simulink model "FuzzyControl"  (Simulink 8.9)
settings: Solver=FixedStepDiscrete  StartTime=0.0  StopTime=inf  FixedStep=0.002  RelTol=1e-3  EnableMultiTasking=on
undefined symbols (not defined in the file or in its folder): DiscIntNeverNeededParam, HIL
libraries: quarc_library x8, fuzblock x1
Description:
  | This example is a simple analog loopback test. It sends a signal to analog output
  | channel #0 and then reads analog input channel #0. Wire analog output #0 to analog
  | input #0 to see the signal on the Scope. Change the amplitude of the signal and see
  | the change occur on the Scope.
settings Model: Creator=drmadill  LastModifiedBy=yettbh  SimulationMode=external  ExtModeTrigDuration=10000
settings SolverCC: PositivePriorityOrder=on
settings OptimizationCC: ExpressionDepthLimit=2147483647  InitFltsAndDblsToZero=on  LifeSpan=auto
settings DebuggingCC: SaveWithParameterizedLinksMsg=none  SolverPrmCheckMsg=warning
settings RTWCC: SystemTargetFile=quarc_win64.tlc  TemplateMakefile=quarc_default_tmf  Description=QUARC Win64 Target
settings STFCustomTargetCC: TargetPreCompLibLocation=C:\PROGRA~3\QUARC\lib\2017a\win64\release  ConcurrentExecutionCompliant=on  SystemTargetFile=quarc_win64.tlc
settings GRTTargetCC: TargetPreCompLibLocation=C:\PROGRA~3\QUARC\lib\2017a\win64\release  ParMdlRefBuildCompliant=off  CompOptLevelCompliant=off  GeneratePreprocessorConditionals=Use local settings  MatFileLogging=off  CPPClassGenCompliant=off  UseToolchainInfoCompliant=off  ExtMode=on  ExtModeMexFile=quarc_comm

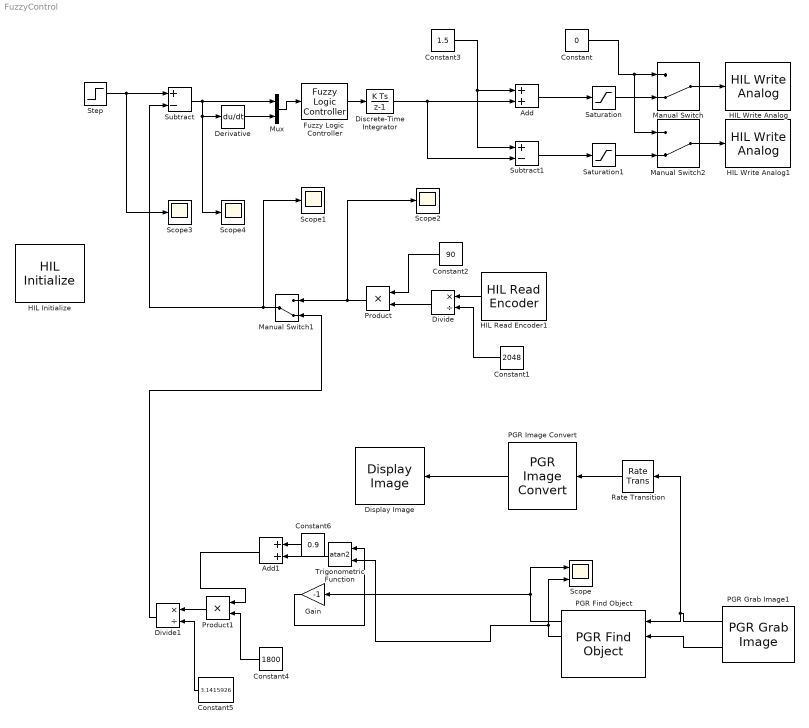
== system FuzzyControl ==
  Add : Sum
  Add1 : Sum
  Constant : Constant  Value=0
  Constant1 : Constant  Value=2048
  Constant2 : Constant  Value=90
  Constant3 : Constant  Value=1.5
  Constant4 : Constant  Value=1800
  Constant5 : Constant  Value=3.1415926
  Constant6 : Constant  Value=0.9
  Derivative : Derivative
  Discrete-Time Integrator : DiscreteIntegrator  SampleTime=0.002  ICPrevOutput=DiscIntNeverNeededParam  ICPrevScaledInput=DiscIntNeverNeededParam
  Display Image : quarc_library/Sinks/Figures/Display Image  figure_mode=Use figure window  figure_tag=figure1  axes_tag=axes1  update_rate=1  initial_position="48  432  563  457"  initial_visibility=off  sample_time=0.1  axes_only=off  orig_size=off
      settings: SourceProductName=QUARC Targets
  Divide : Product  Inputs=*/
  Divide1 : Product  Inputs=*/
  Fuzzy Logic  Controller : fuzblock/Fuzzy Logic  Controller  fis='vision.fis'
  Gain : Gain  Gain=-1
  HIL Initialize : quarc_library/Data Acquisition/Generic/Configuration/HIL Initialize  object_name=HIL-1  board_type=q8  board_number=0  board_options=""  exclusive=off  active=on  hardware_clocks=[0:1]  clock_modes=[0 0]  initial_clock_frequencies=[]  set_clock_params_at_start=on  set_clock_params_at_switch_in=off  set_clock_frequencies_at_start=off  set_clock_frequencies_at_switch_in=off  analog_input_channels=[0:7]  analog_input_configurations=[]  analog_input_maximums=10  analog_input_minimums=-10  set_analog_input_params_at_start=off  set_analog_input_params_at_switch_in=off  analog_output_channels=[0:7]  analog_output_maximums=[10]  analog_output_minimums=[-10]  initial_analog_outputs=[0]  final_analog_outputs=[0]  watchdog_analog_outputs=0  set_analog_output_params_at_start=on  set_analog_output_params_at_switch_in=off  set_analog_outputs_at_start=on  set_analog_outputs_at_switch_in=off  set_analog_outputs_at_terminate=on  set_analog_outputs_at_switch_out=off  set_analog_outputs_on_watchdog=off  digital_input_channels=[]  digital_output_channels=[]  digital_output_configuration=[]  initial_digital_outputs=[1]  final_digital_outputs=[1]  watchdog_digital_outputs=[2]  set_digital_output_params_at_start=off  set_digital_output_params_at_switch_in=off  set_digital_outputs_at_start=on  set_digital_outputs_at_switch_in=off  set_digital_outputs_at_terminate=on  set_digital_outputs_at_switch_out=off  set_digital_outputs_on_watchdog=off  encoder_channels=[0:7]  quadrature=[4]  encoder_filter_frequency=(1/120e-9)/1  initial_encoder_counts=[0]  set_encoder_params_at_start=on  set_encoder_params_at_switch_in=off  set_encoder_counts_at_start=on  set_encoder_counts_at_switch_in=off  pwm_channels=[]  pwm_modes=[0]  pwm_frequency=(1/60e-9)/1024  pwm_configuration=[]  pwm_alignment=[]  pwm_polarity=[]  pwm_leading_deadband=[]  pwm_trailing_deadband=[]  initial_pwm_outputs=[0]  final_pwm_outputs=[0]  watchdog_pwm_outputs=[]  set_pwm_params_at_start=on  set_pwm_params_at_switch_in=off  set_pwm_outputs_at_start=on  set_pwm_outputs_at_switch_in=off  set_pwm_outputs_at_terminate=on  set_pwm_outputs_at_switch_out=off  set_pwm_outputs_on_watchdog=off  other_output_channels=[]  initial_other_outputs=[]  final_other_outputs=[]  watchdog_other_outputs=[]  set_other_outputs_at_start=off  set_other_outputs_at_switch_in=off  set_other_outputs_at_terminate=off  set_other_outputs_at_switch_out=off  set_other_outputs_on_watchdog=off
  HIL Read Encoder1 : quarc_library/Data Acquisition/Generic/Immediate I//O/HIL Read Encoder  object_name=HIL-1  channels=0  sample_time=qc_get_step_size  active=on  vector_output=off  data_type_mode=Inherit via back propagation  data_type=double
  HIL Write Analog : quarc_library/Data Acquisition/Generic/Immediate I//O/HIL Write Analog  object_name=HIL-1  channels=0  sample_time=-1  active=off  vector_input=off
  HIL Write Analog1 : quarc_library/Data Acquisition/Generic/Immediate I//O/HIL Write Analog  object_name=HIL-1  channels=1  sample_time=-1  active=off  vector_input=off
  Manual Switch : ManualSwitch  CurrentSetting=0
  Manual Switch1 : ManualSwitch  CurrentSetting=0
  Manual Switch2 : ManualSwitch  CurrentSetting=0
  Mux : Mux  Inputs=2
  PGR Find Object : quarc_library/Image Processing/Point Grey Research/PGR Find Object  detect_mode=RGB  pixel_format=RGB8  num_objects=1  lum_threshold=70  min_size=100  r_value=50  g_value=70  b_value=70  sample_time=-1
      settings: SourceProductName=QUARC Targets
  PGR Grab Image1 : quarc_library/Devices/Third-Party/Point Grey Research/Cameras/PGR Grab Image  camera_type=FireflyMV  serial_number=-1  video_mode=640x480 RGB  frame_rate=30  left_pos=140  top_pos=20  image_width=440  image_height=440  reset_camera_settings=off  thread_priority=0  sample_time=qc_get_step_size
      settings: SourceProductName=QUARC Targets
  PGR Image Convert : quarc_library/Image Processing/Point Grey Research/PGR Image Convert  pixel_format=RGB8  convert_mode=Matlab RGB  sample_time=0.1
      settings: SourceProductName=QUARC Targets
  Product : Product  RndMeth=Zero
  Product1 : Product  RndMeth=Zero
  Rate Transition : RateTransition
  Saturation : Saturate  UpperLimit=2.5  LowerLimit=0
  Saturation1 : Saturate  UpperLimit=2.5  LowerLimit=0
  Scope : Scope  NumInputPorts=2
  Scope{1..4} (4 alike) : Scope
  Step : Step  Time=3  After=30  SampleTime=0
  Subtract : Sum  Inputs=+-
  Subtract1 : Sum  Inputs=+-
  Trigonometric Function : Trigonometry  Operator=atan2
  wires:
  Subtract/1 -> Mux/1, Scope4/1, Derivative/1
  Step/1 -> Subtract/1, Scope3/1
  Constant3/1 -> Subtract1/1, Add/1
  Add/1 -> Saturation/1
  Subtract1/1 -> Saturation1/1
  Saturation1/1 -> Manual Switch2/2
  Saturation/1 -> Manual Switch/2
  Constant/1 -> Manual Switch/1, Manual Switch2/1
  Manual Switch/1 -> HIL Write Analog/1
  Manual Switch2/1 -> HIL Write Analog1/1
  HIL Read Encoder1/1 -> Divide/1
  Divide/1 -> Product/2
  Constant1/1 -> Divide/2
  Constant2/1 -> Product/1
  Product/1 -> Manual Switch1/1, Scope2/1
  Manual Switch1/1 -> Subtract/2, Scope1/1
  PGR Grab Image1/1 -> PGR Find Object/1, Rate Transition/1
  PGR Grab Image1/2 -> PGR Find Object/2
  PGR Find Object/1 -> Gain/1, Scope/1
  Gain/1 -> Trigonometric Function/1
  PGR Find Object/2 -> Trigonometric Function/2, Scope/2
  Add1/1 -> Product1/1
  Constant4/1 -> Product1/2
  Product1/1 -> Divide1/1
  Constant5/1 -> Divide1/2
  PGR Image Convert/1 -> Display Image/1
  Rate Transition/1 -> PGR Image Convert/1
  Fuzzy Logic  Controller/1 -> Discrete-Time Integrator/1
  Discrete-Time Integrator/1 -> Subtract1/2, Add/2
  Derivative/1 -> Mux/2
  Mux/1 -> Fuzzy Logic  Controller/1
  Divide1/1 -> Manual Switch1/2
  Trigonometric Function/1 -> Add1/2
  Constant6/1 -> Add1/1
